simulink model "Simulacion"  (R2022b)
settings: Solver=ode4  StartTime=0.0  StopTime=30  FixedStep=0.0001  RelTol=1e-3
undefined symbols (not defined in the file): A, B, k1, k2, ne, nq, P, W1_0, W2_0
settings Model: Creator=raul  LastModifiedBy=raul

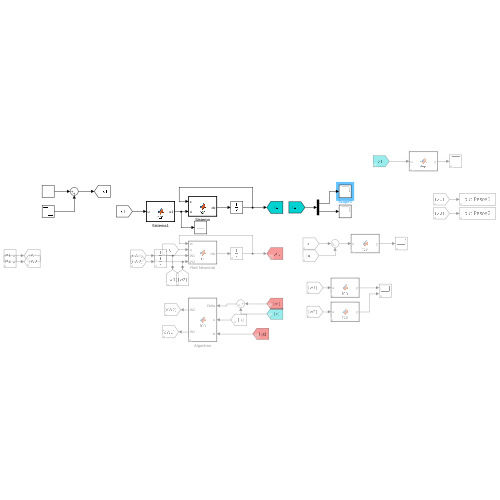
[thumbnail: Simulink's stored preview of the top-level diagram]
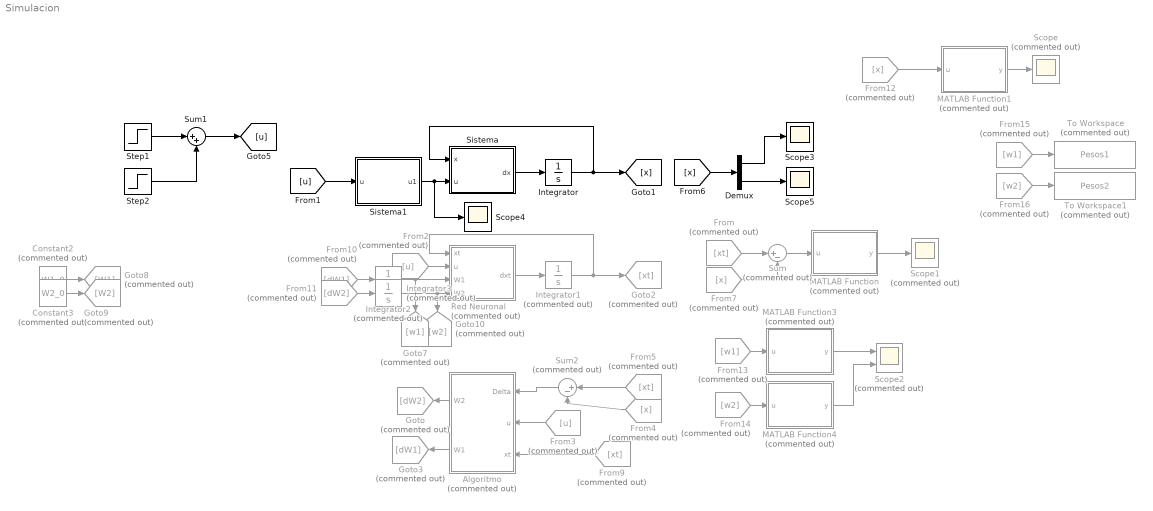
== system Simulacion ==
  Algoritmo : MATLAB Function  Commented=on  TreatAsAtomicUnit=on
  Constant2 : Constant  Commented=on  Value=W1_0
  Constant3 : Constant  Commented=on  Value=W2_0
  Demux : Demux  Outputs=2
  From : From  Commented=on  GotoTag=xt
  From10 : From  Commented=on  GotoTag=dW1
  From11 : From  Commented=on  GotoTag=dW2
  From12 : From  Commented=on  GotoTag=x
  From13 : From  Commented=on  GotoTag=w1
  From14 : From  Commented=on  GotoTag=w2
  From15 : From  Commented=on  GotoTag=w1
  From16 : From  Commented=on  GotoTag=w2
  From2 : From  Commented=on  GotoTag=u
  From3 : From  Commented=on  GotoTag=u
  From4 : From  Commented=on  GotoTag=x
  From5 : From  Commented=on  GotoTag=xt
  From7 : From  Commented=on  GotoTag=x
  From9 : From  Commented=on  GotoTag=xt
  Goto : Goto  Commented=on  GotoTag=dW2
  Goto10 : Goto  Commented=on  GotoTag=w2
  Goto2 : Goto  Commented=on  GotoTag=xt
  Goto3 : Goto  Commented=on  GotoTag=dW1
  Goto7 : Goto  Commented=on  GotoTag=w1
  Goto8 : Goto  Commented=on  GotoTag=W1
  Goto9 : Goto  Commented=on  GotoTag=W2
  Integrator : Integrator  InitialCondition=zeros(2*ne,1)
  Integrator1 : Integrator  Commented=on  InitialCondition=zeros(2*nq,20)
  Integrator2 : Integrator  Commented=on  InitialCondition=W1_0
  Integrator3 : Integrator  Commented=on  InitialCondition=W2_0
  MATLAB Function : MATLAB Function  Commented=on  TreatAsAtomicUnit=on
  MATLAB Function1 : MATLAB Function  Commented=on  TreatAsAtomicUnit=on
  MATLAB Function3 : MATLAB Function  Commented=on  TreatAsAtomicUnit=on
  MATLAB Function4 : MATLAB Function  Commented=on  TreatAsAtomicUnit=on
  Red Neuronal : MATLAB Function  Commented=on  TreatAsAtomicUnit=on
  Scope : Scope  Commented=on
  Scope1 : Scope  Commented=on
  Scope2 : Scope  Commented=on  NumInputPorts=2
  Scope3 : Scope
  Scope4 : Scope
  Scope5 : Scope
  Sistema : MATLAB Function  TreatAsAtomicUnit=on
  Sistema1 : MATLAB Function  TreatAsAtomicUnit=on
  Step1 : Step  After=100  SampleTime=0
  Step2 : Step  Time=1.3  After=-100  SampleTime=0
  Sum : Sum  Commented=on  Inputs=|+-
  Sum1 : Sum  Inputs=|++
  Sum2 : Sum  Commented=on  Inputs=|+-
  To Workspace : ToWorkspace  Commented=on  VariableName=Pesos1  SampleTime=-1
  To Workspace1 : ToWorkspace  Commented=on  VariableName=Pesos2  SampleTime=-1
  wires:
  Step2/1 -> Sum1/2
  Step1/1 -> Sum1/1
  Sistema/1(dx) -> Integrator/1
  Integrator/1 -> [x], Sistema/1(x)
  From/1 -> Sum/1
  From7/1 -> Sum/2
  Red Neuronal/1(dxt) -> Integrator1/1
  Integrator1/1 -> Goto2/1, Red Neuronal/1(xt)
  Sum1/1 -> [u]
  From2/1 -> Red Neuronal/2(u)
  From3/1 -> Algoritmo/2(u)
  Sum2/1 -> Algoritmo/1(Delta)
  From4/1 -> Sum2/2
  From5/1 -> Sum2/1
  Algoritmo/1(W2) -> Goto/1
  Algoritmo/2(W1) -> Goto3/1
  From9/1 -> Algoritmo/3(xt)
  Constant2/1 -> Goto8/1
  Constant3/1 -> Goto9/1
  Sum/1 -> MATLAB Function/1(u)
  MATLAB Function/1(y) -> Scope1/1
  MATLAB Function1/1(y) -> Scope/1
  From12/1 -> MATLAB Function1/1(u)
  Integrator3/1 -> Goto10/1, Red Neuronal/4(W2)
  Integrator2/1 -> Goto7/1, Red Neuronal/3(W1)
  From11/1 -> Integrator3/1
  From10/1 -> Integrator2/1
  From13/1 -> MATLAB Function3/1(u)
  MATLAB Function3/1(y) -> Scope2/1
  From14/1 -> MATLAB Function4/1(u)
  MATLAB Function4/1(y) -> Scope2/2
  From16/1 -> To Workspace1/1
  From15/1 -> To Workspace/1
  Sistema1/1(u1) -> Scope4/1, Sistema/2(u)
  [u] -> Sistema1/1(u)
  [x] -> Demux/1
  Demux/1 -> Scope3/1
  Demux/2 -> Scope5/1

== matlab function Simulacion/Algoritmo ==
  data: W2 output; Delta input; P parameter; u input; W1 output; k1 parameter; k2 parameter; xt input
function [W2,W1] = fcn(Delta,P,u, k1, k2,xt)


W1=-k1*P*Delta*sigmoid(1,xt)';
W2=-k2*P*Delta*sigmoid(1,xt)'*u;


% function [du, dW, dV] = DNN(u, us, W1, V1, h)
% 	Delta   = u - us;
% 	sigma   = sigmoid(1,V1*u);
% 	D_sigma = diag(sigma.*(1-sigma));
% 	%
% 	dW      = h*(-K1NN*PNN*Delta*sigma' + K1NN*PNN*Delta*u'*(V1-V0NN)'*D_sigma);
% 	dV		= h*(-K2NN*D_sigma'*W1'*PNN*Delta*u' - lNN/2*K2NN*LambdaNN*(V1-V0NN)*(u*u'));
% 	du		= h*(ANN*u + W1*sigma);
% end


function s = sigmoid(b,x)
   s = 1./(1+exp(-b*x)); 
end

end

== matlab function Simulacion/Red Neuronal ==
  data: xt input; u input; dxt output; W1 input; A parameter; W2 input
function dxt = fcn(xt, u, W1, A, W2)

dxt = A*xt+W1*sigmoid(1,xt)+W2*sigmoid(1,xt)*u;


function s = sigmoid(b,x)
   s = 1./(1+exp(-b*x)); 
end

end

== matlab function Simulacion/Sistema ==
  data: x input; u input; dx output; A parameter; B parameter
function dx = fcn(x,u,A, B)%add Bw,w

dx = A*x+B*u;

%dx = A*x+B(:,f)*u+Bw*w;

== matlab function Simulacion/MATLAB Function ==
  data: u input; y output
function y = fcn(u)

y = u(:,20);

== matlab function Simulacion/MATLAB Function1 ==
  data: u input; y output; f parameter
function y = fcn(u,f)

y = u(:,f);

== matlab function Simulacion/MATLAB Function3 ==
  data: u input; y output; f parameter
function y = fcn(u,f)

y = u(:,f);

== matlab function Simulacion/MATLAB Function4 ==
  data: u input; y output; f parameter
function y = fcn(u,f)

y = u(:,f);

== matlab function Simulacion/Sistema1 ==
  data: u1 output; u input
function u1 = fcn(u)%add Bw,w

u1=[0;0;0;0;0;0;0;0;0;0;0;u;0;0;0;0;0;0;0;0];
